simulink model "nav_leha19b"  (R2019b)
settings: Solver=FixedStepDiscrete  StartTime=0.0  StopTime=2500  FixedStep=dT  RelTol=1e-3
values from neighbouring files (symbols this model uses):
  al_gp_M = k    (= 2)    [gnss_data_orig.m]
  al_gp_max = 15    [model_nav_system_flight_simulation_orig.m]
  al_gp_mu = 3.986004418E+14    (= 398600441800000)    [gnss_data_orig.m]
  al_gp_resolution = 1000    [gnss_data_orig.m]
  al_gp_t0 = gnss_strings_2(1,4)    [gnss_data_orig.m]
  dT = 1    [model_nav_system_flight_simulation_orig.m]
  mean_p_ion = 1.3    [model_nav_system_flight_simulation_orig.m]
  mean_p_trop = 0.3    [model_nav_system_flight_simulation_orig.m]
  P0_b_g = zeros(23,23)    [model_nav_system_flight_simulation_orig.m]
  P_b = zeros(21, 21)    [model_nav_system_flight_simulation_orig.m]
  R_a = 6378136    [model_nav_system_flight_simulation_orig.m]
  R_betta = 0.0053171    [model_nav_system_flight_simulation_orig.m]
  R_betta1 = 71 * 10^-7    (= 7.1e-06)    [model_nav_system_flight_simulation_orig.m]
  R_e2 = 0    [model_nav_system_flight_simulation_orig.m]
  R_ge = 9.78049    [model_nav_system_flight_simulation_orig.m]
  R_q = 0.00346775    [model_nav_system_flight_simulation_orig.m]
  R_u = 7.292115*10^(-5)    (= 7.292115e-05)    [model_nav_system_flight_simulation_orig.m]
  sigma_error_acs0 = [SKO_del_n_x SKO_del_n_y SKO_del_n_z]    [model_nav_system_flight_simulation_orig.m]
  sigma_error_DUS0 = [SKO_del_Omega_x SKO_del_Omega_y SKO_del_Omega_z]    [model_nav_system_flight_simulation_orig.m]
  sigma_gnss0 = SKO_p_del_T + SKO_p_del_t + mean_p_ion + mean_p_trop + SKO_p_mnogoluch + SKO_p_noise    (= 5.61)    [model_nav_system_flight_simulation_orig.m]
  SKO_p_del_T = 3    [model_nav_system_flight_simulation_orig.m]
  SKO_p_del_t = 0.01    [model_nav_system_flight_simulation_orig.m]
  SKO_p_mnogoluch = 0.5    [model_nav_system_flight_simulation_orig.m]
  SKO_p_noise = 0.5    [model_nav_system_flight_simulation_orig.m]
  tr_H = flight_mission(3,1)    [model_nav_system_flight_simulation_orig.m]
  W = W'    [model_nav_system_flight_simulation_orig.m]
  X0 = X0'    [model_nav_system_flight_simulation_orig.m]
  X0_b_g = X0_b_g * 0    [model_nav_system_flight_simulation_orig.m]
undefined symbols (not defined in the file or in its folder): al_gp_e, al_gp_health, al_gp_i, al_gp_lan, al_gp_m0, al_gp_sqrt_a, al_gp_w, sigma_error_D_p, sigma_error_D_p1, sigma_gnss0_0, tr_course, tr_fi, tr_la, tr_pitch, tr_roll, tr_V_E, tr_V_H, tr_V_N, tr_X_dgsk, tr_Y_dgsk, tr_Z_dgsk
libraries: simulink_extras x8
(part 3 of 3)

== matlab function nav_leha19b/Алгоритм ССК + UKF/MATLAB Function2 ==
  data: P input; P output; x input; x output; z_k input; F input; H input; G input; R_k input; Q_km1 input; PP output; dt input
function [P, x, PP] = ukf_2(P, x, z_k, F, H, G, R_k, Q_km1, dt)
    
    % раpмерности
    nx = length(x);         
    nq = size(Q_km1, 1);    
    nz = size(R_k, 1);      
    L  = nx + nq + nz;      
    ns = 2 * L + 1;  %число всех сигма точек 

    f = @(X, W) (eye(nx) + F*dt + (F*dt)^2./2) * X + ((eye(nx)+F*dt/2)*G*dt) * W;
    h = @(X, satelite_errors) H * X - satelite_errors; 
	% альфа бетта каппа
    alpha = 0.001;
    beta  = 2;
    kappa = 0;
    
    % вычисленеи весов
    lambda = alpha ^2 * (L + kappa) - L;
    gamma  = sqrt(L + lambda);
    W_m_0  = lambda / (L + lambda);
    W_c_0  = W_m_0 + 1 - alpha^2 + beta;
    W_i    = 1/(2*(L + lambda));
    % дополненная система
    P_a     = blkdiag(P, Q_km1, R_k); %располагаем матрицы по диагонали
    x_a_km1 = [x; zeros(nq, 1); zeros(nz, 1)]; %дополняем вектор состояния
    
    % сигматочечное разложение
%     [u, s] = svd(P_a);
%     gamma_sqrt_P_a = gamma * u * sqrt(s);
%     e = repmat(x_a_km1, 1, L);
%     X_a_km1 = [x_a_km1, ...
%                repmat(x_a_km1, 1, L) + gamma_sqrt_P_a, ...
%                repmat(x_a_km1, 1, L) - gamma_sqrt_P_a];
    gamma_sqrt_P_a = gamma*chol(P_a)';
    e = chol(P_a);
    X_a_km1 = [x_a_km1,...
        repmat(x_a_km1, 1, L) + gamma_sqrt_P_a, ...
        repmat(x_a_km1, 1, L) - gamma_sqrt_P_a,];
    Z_kkm1   = zeros(nz, ns);
    X_x_kkm1 = zeros(nx, ns);
    for sp = 1:ns
        X_x_kkm1(:, sp) = f(X_a_km1(1:nx, sp), X_a_km1(nx+1:nx+nq, sp));            
        Z_kkm1(:, sp)   = h(X_x_kkm1(1:nx, sp), X_a_km1(nx+nq+1:nx+nq+nz, sp));                   
    end
    
    x_kkm1 = W_m_0 * X_x_kkm1(:, 1) + W_i * sum(X_x_kkm1(:, 2:end), 2);
    z_kkm1 = W_m_0 * Z_kkm1(:, 1)   + W_i * sum(Z_kkm1(:, 2:end), 2);

%     X_x_kkm1 = bsxfun(@minus, X_x_kkm1, x_kkm1);
%     Z_kkm1   = bsxfun(@minus, Z_kkm1, z_kkm1);

    X_x_kkm1 = X_x_kkm1 - x_kkm1;
    Z_kkm1   = Z_kkm1 - z_kkm1;
    
    P_kkm1 =   (W_c_0 * X_x_kkm1(:, 1)) * X_x_kkm1(:, 1).' ...
             + W_i * (X_x_kkm1(:, 2:end) * X_x_kkm1(:, 2:end).');

    P_zz =   (W_c_0 * Z_kkm1(:, 1)) * Z_kkm1(:, 1).' ...
           + W_i * (Z_kkm1(:, 2:end) * Z_kkm1(:, 2:end).');
    
    P_xz =   (W_c_0 * X_x_kkm1(:, 1)) * Z_kkm1(:, 1).' ...
           + W_i * (X_x_kkm1(:, 2:end) * Z_kkm1(:, 2:end).');
       
    K = P_xz / P_zz;
    x = x_kkm1 + K * (z_k - Z_kkm1);
    P = P_kkm1 - K * P_zz * K.';
    PP = zeros(21,1);
    for i = 1:1:nx
        PP (i) = sqrt(P(i,i));
    end
end

== matlab function nav_leha19b/Сравнение ССK  и CCK + UKF/MATLAB Function ==
  data: real_data input; plot1 output; estimate input; plot2 output
function [plot1, plot2] = fcn(real_data, estimate)
plot1 = abs(real_data(1));
plot2 = abs(estimate(1));

== matlab function nav_leha19b/Сравнение ССK  и CCK + UKF/MATLAB Function1 ==
  data: real_data input; plot1 output; estimate input; plot2 output
function [plot1, plot2] = fcn(real_data, estimate)
plot1 = abs(real_data(1));
plot2 = abs(estimate(1));

== matlab function nav_leha19b/Алгоритм ЖСК БИНС + ГНСС + UKF/MATLAB Function ==
  settings: updateMethod=DISCRETE  sampleTime=dT
  data: tr_la input; tr_fi input; tr_H input; tr_V_H input; R1 input; ro1 input; H_b_g output size=[2 * al_gp_max, 23]; ro2 input; R_a input; R_e2 input; b_D_p input; pos_x_dgks input; pos_y_dgks input; pos_z_dgks input; b_X_dgsk input; b_Y_dgsk input; b_Z_dgsk input; Omega_id_geogr input; see_flag input; al_gp_max input
function H_b_g = H_b_gp(tr_la, tr_fi, tr_H, tr_V_H, R1, ro1, ro2, R_a, R_e2, b_D_p, pos_x_dgks, pos_y_dgks, pos_z_dgks, b_X_dgsk, b_Y_dgsk, b_Z_dgsk, Omega_id_geogr, see_flag, al_gp_max)
    persistent i j m
    m = sum(see_flag);
    b_la = tr_la;
    b_fi = tr_fi;
    b_H = tr_H;
    b_V_H = tr_V_H;

    Omega_E = Omega_id_geogr(1);
    Omega_N = Omega_id_geogr(2);
    Omega_H = Omega_id_geogr(3);

    i = int8(1);
    j = int8(1);
    
    H_b_g = zeros(2 * al_gp_max, 23);

    while j <= 31
        if see_flag(j) > 0.5
            dR1_db_fi = (R_a * R_e2 * cos(b_fi) * sin(b_fi)) / (( 1 - R_e2 * ((sin(b_fi)) ^ 2)) ^ (3/2));
            
            %Rtp = sin(b_fi) * (R1 + b_H) - cos(b_fi) * dR1_db_fi;
            
            dp_dfi = (1 / b_D_p(j)) * ...
                    ((pos_x_dgks(j) - b_X_dgsk) * (- cos(b_la) * cos(b_fi) * dR1_db_fi + (R1 + b_H) * cos(b_la) * sin(b_fi)) + ...
                     (pos_y_dgks(j) - b_Y_dgsk) * (- sin(b_la) * cos(b_fi) * dR1_db_fi + (R1 + b_H) * sin(b_la) * sin(b_fi)) + ...
                     (pos_z_dgks(j) - b_Z_dgsk) * ( - (1 - R_e2) * sin(b_fi) * dR1_db_fi - ((1 - R_e2) * R1 + b_H) * cos(b_fi)));
            
            dp_dH  = (-1 / b_D_p(j)) * (cos(b_fi) * cos(b_la) * (pos_x_dgks(j) - b_X_dgsk) + ...
                     cos(b_fi) * sin(b_la) * (pos_y_dgks(j) - b_Y_dgsk) + ...
                     sin(b_fi) * (pos_z_dgks(j) - b_Z_dgsk));
                 
            H_b_g(i,1) = (1 / b_D_p(j)) * (sin(b_la) * ... 
                         (pos_x_dgks(j) - b_X_dgsk) - cos(b_la) * (pos_y_dgks(j) - b_Y_dgsk));
            H_b_g(i,2) = (1 / ro1) * dp_dfi;
            H_b_g(i,3) = dp_dH;
            H_b_g(i,20) = -1;
            
            i = i + 1;
            j = j + 1;
        else
            j = j + 1;
        end
    end
    i = int8(m + 1 + (al_gp_max - m));
    j = int8(1);
    while j <= 31
        if see_flag(j) > 0.5
            dp1_db_V_E = (1 / b_D_p(j)) * (sin(b_la) * (pos_x_dgks(j) - b_X_dgsk) - ...
            cos(b_la) * (pos_y_dgks(j) - b_Y_dgsk)); %* del_b_V_E;
        
            dp1_db_V_N = (1 / b_D_p(j)) * (cos(b_la) * sin(b_fi) * (pos_x_dgks(j) - b_X_dgsk) + ...
            sin(b_la) * sin(b_fi) * (pos_y_dgks(j) - b_Y_dgsk) - cos(b_fi) * (pos_z_dgks(j) - b_Z_dgsk));% * del_b_V_N;
            
            dp1_db_V_H = (- 1 / b_D_p(j)) * (cos(b_la) * cos(b_fi) * (pos_x_dgks(j) - b_X_dgsk) + ...
            sin(b_la) * cos(b_fi) * (pos_y_dgks(j) - b_Y_dgsk) + sin(b_fi) * (pos_z_dgks(j) - b_Z_dgsk));% * del_b_V_H;
        
            H_b_g(i,1) = - ((b_V_H / ro2) + Omega_E * tan(b_fi)) * dp1_db_V_E;
            H_b_g(i,2) = - Omega_H * dp1_db_V_E - (b_V_H / ro1) * dp1_db_V_N;
            H_b_g(i,3) = Omega_N * dp1_db_V_E - Omega_E * dp1_db_V_N;
            H_b_g(i,4) = dp1_db_V_E;
            H_b_g(i,5) = dp1_db_V_N;
            H_b_g(i,6) = dp1_db_V_H;
            H_b_g(i,23) = 1;
            
            i = i + 1;
            j = j + 1;
        else
            j = j + 1;
        end
    end

end

== matlab function nav_leha19b/Алгоритм ЖСК БИНС + ГНСС + UKF/MATLAB Function1 ==
  data: rate_X input; Z_b_g_ output size=[30,1]; del_D_p input; D_p input; D1_p input; al_gp_max input
function Z_b_g_ = h(rate_X, del_D_p, D_p, D1_p, al_gp_max)



n = 1;
if n == 1
    Z_b_g_ = zeros(2 * al_gp_max, 1);
    n = n+1;
end
b_D_p = zeros(31,1);
b_D1_p = zeros(31,1);

for i = 1:1:31
    if see_flag(i) > 0.5
        B = [ -sin(tr_la), cos(tr_la), 0;
            -cos(tr_la) * sin(tr_fi), -sin(tr_la) * sin(tr_fi), cos(tr_fi);
            cos(tr_la) * cos(tr_fi), sin(tr_la) * cos(tr_fi), sin(tr_fi)];
        b_V = (B') * [tr_V_E + rate_X(4) - ( (tr_V_H ./ ro2) + Omega_id_geogr(1) .* tan(tr_fi) ) .* rate_X(1) - Omega_id_geogr(3) .* rate_X(2); tr_V_N + rate_X(5) - ( tr_V_H ./ ro1 ) .* rate_X(1); tr_V_H + rate_X(6)];

        b_D_p(i) = sqrt ( (pos_x_dgsk(i) - (tr_H + rate_X(3) + R_a / sqrt(1 - R_e2 * (sin(tr_fi) ^ 2))) * cos(tr_fi + rate_X(2) ./ ro1) * cos(tr_la + rate_X(1) ./ ( ro2 .* cos(tr_fi) ))).^2 + ...
            (pos_y_dgsk(i) - (tr_H + rate_X(3) + R_a / sqrt(1 - R_e2 * (sin(tr_fi) ^ 2))) * cos(tr_fi + rate_X(2) ./ ro1) * sin(tr_la + rate_X(1) ./ ( ro2 .* cos(tr_fi) ))).^2 + ...
            (pos_z_dgsk(i) - ((1 - R_e2) * R_a / sqrt(1 - R_e2 * (sin(tr_fi) ^ 2)) + tr_H + rate_X(3)) * sin(tr_fi + rate_X(2) ./ ro1)).^2);
        b_D1_p(i) = (((pos_x_dgsk(i) - (tr_H + rate_X(3) + R_a / sqrt(1 - R_e2 * (sin(tr_fi) ^ 2))) * cos(tr_fi + rate_X(2) ./ ro1) * cos(tr_la + rate_X(1) ./ ( ro2 .* cos(tr_fi) ))) .* (vel_x_dgsk(i) - b_V(1))) + ...
            ( (pos_y_dgsk(i) - (tr_H + rate_X(3) + R_a / sqrt(1 - R_e2 * (sin(tr_fi) ^ 2))) * cos(tr_fi + rate_X(2) ./ ro1) * sin(tr_la + rate_X(1) ./ ( ro2 .* cos(tr_fi) ))) .* (vel_y_dgsk(i) - b_V(2))) + ...
            ( (pos_z_dgsk(i) - ((1 - R_e2) * R_a / sqrt(1 - R_e2 * (sin(tr_fi) ^ 2)) + tr_H + rate_X(3)) * sin(tr_fi + rate_X(2) ./ ro1)) .* (vel_z_dgsk(i) - b_V(3)))) ./ b_D_p(i);

    else
        b_D_p(i) = NaN;
        b_D1_p(i) = NaN;
    end
end
m = sum(see_flag);
i = 1;
for j = 1:1:31
    if see_flag(j) == 1
        Z_b_g_(i) = b_D_p(j) - D_p(j);
        i = i + 1;
    end
end
i = m + 1 + (al_gp_max - m);
for j = 1:1:31
    if see_flag(j) == 1
        Z_b_g_(i) = b_D1_p(j) - D1_p(j);
        i = i + 1;
    end
end
Z_b_g_ = Z_b_g_ + del_D_p;
end

== matlab function nav_leha19b/Алгоритм ЖСК БИНС + ГНСС/MATLAB Function2 ==
  data: X_diff input; X_feedback output; X_b input
function X_feedback = fcn(X_diff, X_b)
X_feedback = X_b;
X_feedback(1:2) = X_diff(1:2);
X_feedback(4:5) = X_diff(4:5);
X_feedback(7:21) = X_diff(7:21);
end

== matlab function nav_leha19b/Алгоритм ЖСК БИНС + ГНСС + UKF/MATLAB Function2 ==
  data: X_diff input; X_b input; X_feedback output
function X_feedback = fcn(X_diff, X_b)
X_feedback = X_b;
X_feedback(1:2) = X_diff(1:2);
X_feedback(4:5) = X_diff(4:5);
X_feedback(7:21) = X_diff(7:21);
end

== matlab function nav_leha19b/Алгоритм ЖСК БИНС + ГНСС + UKF/MATLAB Function3 ==
  data: F_b input size=[21,21]; G_b input; F_b_g output size=[23,23]; G_b_g output
function [F_b_g, G_b_g]  = fcn(F_b, G_b)

    F_b_g = zeros(23,23);
    F_b_g(1:21, 1:21) = F_b;

    G_b_g = zeros(23,6);
    G_b_g(1:21, 1:6) = G_b;
    
end

== matlab function nav_leha19b/pseudorange/MATLAB Function4 ==
  data: El input; HDOP output; az input; see_flag input; VDOP output; PDOP output; TDOP output; al_gp_max input
function [HDOP, VDOP, PDOP, TDOP] = fcn(El, az, see_flag, al_gp_max)
DOP_A = zeros(al_gp_max,4);

persistent i k
k = 1;
for i = 1:31
    if see_flag(i) > 0.5
        DOP_A(k,1) = - cos(El(i))*cos(az(i));
        DOP_A(k,2) = - cos(El(i))*sin(az(i));
        DOP_A(k,3) = - sin(El(i));
        DOP_A(k,4) = 1;
        k = k + 1;
    end
end
DOP_H = (DOP_A'*DOP_A)^(-1);
HDOP = sqrt(DOP_H(1,1) + DOP_H(2,2));
VDOP = sqrt(DOP_H(3,3));
PDOP = sqrt(DOP_H(1,1) + DOP_H(2,2) + DOP_H(3,3));
TDOP = sqrt(DOP_H(4,4));

== matlab function nav_leha19b/Алгоритм ЖСК БИНС + ГНСС + UKF/MATLAB Function4 ==
  settings: updateMethod=DISCRETE  sampleTime=dT
  data: P input; P output; x input; z_k input; F input; G input; R_k input; Q_km1 input; dt input; x output; x_21 output size=21; PP output size=[23]; x12 output size=2; pos_x_dgsk input; pos_y_dgsk input; pos_z_dgsk input; vel_x_dgsk input; vel_y_dgsk input; vel_z_dgsk input; see_flag input; tr_fi input; tr_la input; tr_H input; tr_V_E input; tr_V_N input; tr_V_H input; ro1 input; ro2 input; R_a input; R_e2 input; al_gp_max input; D_p input; Omega_id_geogr input; D1_p input; e output size=[1,1]; l output size=[1,1]
function [P, x, x_21, PP, x12, e, l] = ukf_2(P, x, z_k, F, G, R_k, Q_km1, dt, pos_x_dgsk, pos_y_dgsk, pos_z_dgsk, vel_x_dgsk, vel_y_dgsk, vel_z_dgsk, see_flag, tr_fi, tr_la, tr_H, tr_V_E, tr_V_N, tr_V_H, ro1, ro2, R_a, R_e2, al_gp_max, D_p, Omega_id_geogr, D1_p)

    function Z_b_g_ = h(rate_X, del_D_p)
        n = 1;
        if n == 1
            Z_b_g_ = zeros(2 * al_gp_max, 1);
            n = n+1;
        end
        b_D_p = zeros(31,1);
        b_D1_p = zeros(31,1);

        for i = 1:1:31
            if see_flag(i) > 0.5
                B = [ -sin(tr_la), cos(tr_la), 0;
                    -cos(tr_la) * sin(tr_fi), -sin(tr_la) * sin(tr_fi), cos(tr_fi);
                    cos(tr_la) * cos(tr_fi), sin(tr_la) * cos(tr_fi), sin(tr_fi)];
                b_V = (B') * [tr_V_E + rate_X(4) - ( (tr_V_H ./ ro2) + Omega_id_geogr(1) .* tan(tr_fi) ) .* rate_X(1) - Omega_id_geogr(3) .* rate_X(2); tr_V_N + rate_X(5) - ( tr_V_H ./ ro1 ) .* rate_X(1); tr_V_H + rate_X(6)];

                b_D_p(i) = sqrt ( (pos_x_dgsk(i) - (tr_H + rate_X(3) + R_a / sqrt(1 - R_e2 * (sin(tr_fi) ^ 2))) * cos(tr_fi + rate_X(2) ./ ro1) * cos(tr_la + rate_X(1) ./ ( ro2 .* cos(tr_fi) ))).^2 + ...
                    (pos_y_dgsk(i) - (tr_H + rate_X(3) + R_a / sqrt(1 - R_e2 * (sin(tr_fi) ^ 2))) * cos(tr_fi + rate_X(2) ./ ro1) * sin(tr_la + rate_X(1) ./ ( ro2 .* cos(tr_fi) ))).^2 + ...
                    (pos_z_dgsk(i) - ((1 - R_e2) * R_a / sqrt(1 - R_e2 * (sin(tr_fi) ^ 2)) + tr_H + rate_X(3)) * sin(tr_fi + rate_X(2) ./ ro1)).^2);
                b_D1_p(i) = (((pos_x_dgsk(i) - (tr_H + rate_X(3) + R_a / sqrt(1 - R_e2 * (sin(tr_fi) ^ 2))) * cos(tr_fi + rate_X(2) ./ ro1) * cos(tr_la + rate_X(1) ./ ( ro2 .* cos(tr_fi) ))) .* (vel_x_dgsk(i) - b_V(1))) + ...
                ( (pos_y_dgsk(i) - (tr_H + rate_X(3) + R_a / sqrt(1 - R_e2 * (sin(tr_fi) ^ 2))) * cos(tr_fi + rate_X(2) ./ ro1) * sin(tr_la + rate_X(1) ./ ( ro2 .* cos(tr_fi) ))) .* (vel_y_dgsk(i) - b_V(2))) + ...
                ( (pos_z_dgsk(i) - ((1 - R_e2) * R_a / sqrt(1 - R_e2 * (sin(tr_fi) ^ 2)) + tr_H + rate_X(3)) * sin(tr_fi + rate_X(2) ./ ro1)) .* (vel_z_dgsk(i) - b_V(3)))) ./ b_D_p(i);

            else
                b_D_p(i) = NaN;
                b_D1_p(i) = NaN;
            end
        end
        m = sum(see_flag);
        i = 1;
        for j = 1:1:31
            if see_flag(j) == 1
                Z_b_g_(i) = b_D_p(j) - D_p(j);
                i = i + 1;
            end
        end
        i = m + 1 + (al_gp_max - m);
        for j = 1:1:31
            if see_flag(j) == 1
                Z_b_g_(i) = b_D1_p(j) - D1_p(j);
                i = i + 1;
            end
        end
       Z_b_g_ = Z_b_g_ + del_D_p;
    end

% размерности
nx = length(x);
nq = size(Q_km1, 1);
nz = size(R_k, 1);
L  = nx + nq + nz;
ns = 2 * L + 1;  %число всех сигма точек

f = @(X, W) (eye(nx) + F*dt + (F*dt)^2./2) * X + ((eye(nx)+F*dt/2)*G*dt) * W;
%     h = @(X, satelite_errors) H * X;% - satelite_errors;
% альфа бетта каппа
alpha = 0.001;
beta  = 2;
kappa = 3 - nx;

% вычисленеи весов
lambda = alpha ^2 * (L + kappa) - L;
gamma  = sqrt(L + lambda);
W_m_0  = lambda / (L + lambda);
W_c_0  = W_m_0 + 1 - alpha^2 + beta;
W_i    = 1/(2*(L + lambda));
% дополненная система
P_a     = blkdiag(P, Q_km1, R_k); %располагаем матрицы по диагонали
x_a_km1 = [x; zeros(nq, 1); zeros(nz, 1)]; %дополняем вектор состояния

gamma_sqrt_P_a = gamma*chol(P_a)';
X_a_km1 = [x_a_km1,...
    repmat(x_a_km1, 1, L) + gamma_sqrt_P_a, ...
    repmat(x_a_km1, 1, L) - gamma_sqrt_P_a,];
Z_kkm1   = zeros(nz, ns);
X_x_kkm1 = zeros(nx, ns);
for sp = 1:ns
    X_x_kkm1(:, sp) = f(X_a_km1(1:nx, sp), X_a_km1(nx+1:nx+nq, sp));
    Z_kkm1(:, sp)   = h(X_x_kkm1(1:nx, sp), X_a_km1(nx+nq+1:nx+nq+nz, sp));
end

x_kkm1 = W_m_0 * X_x_kkm1(:, 1) + W_i * sum(X_x_kkm1(:, 2:end), 2);
z_kkm1 = W_m_0 * Z_kkm1(:, 1)   + W_i * sum(Z_kkm1(:, 2:end), 2);

%     X_x_kkm1 = bsxfun(@minus, X_x_kkm1, x_kkm1);
%     Z_kkm1   = bsxfun(@minus, Z_kkm1, z_kkm1);

X_x_kkm1 = X_x_kkm1 - x_kkm1;
Z_kkm1   = Z_kkm1 - z_kkm1;

P_kkm1 =   (W_c_0 * X_x_kkm1(:, 1)) * X_x_kkm1(:, 1).' ...
    + W_i * (X_x_kkm1(:, 2:end) * X_x_kkm1(:, 2:end).');

P_zz =   (W_c_0 * Z_kkm1(:, 1)) * Z_kkm1(:, 1).' ...
    + W_i * (Z_kkm1(:, 2:end) * Z_kkm1(:, 2:end).');

P_xz =   (W_c_0 * X_x_kkm1(:, 1)) * Z_kkm1(:, 1).' ...
    + W_i * (X_x_kkm1(:, 2:end) * Z_kkm1(:, 2:end).');

K = P_xz / P_zz;
e = z_k(1,1);
size(e);

l = z_kkm1(1,1);
size(l);
x = x_kkm1 + K * (z_k - z_kkm1);
P = P_kkm1 - K * P_zz * K.';
PP = zeros(nx,1);
for ii = 1:1:nx
    PP(ii) = sqrt(P(ii,ii));
end
x_21 = x(1:21);
x12 = x(1:2);
% ZZ = h(X, 0);
% size(ZZ)
end

== matlab function nav_leha19b/Алгоритм ЖСК БИНС + ГНСС + UKF/MATLAB Function5 ==
  settings: updateMethod=DISCRETE  sampleTime=dT
  data: sigma_error_D_p input; Rv_b_g output size=[2 * al_gp_max, 2 * al_gp_max]; sigma_error_D_p1 input; sigma_error_DUS input; sigma_error_acs input; SKO_gnss0 input; sigma_error_DUS0 input; sigma_error_acs0 input; dt input; Q_W output; T input; see_flag input; al_gp_max input
function [Rv_b_g, Q_W] = fcn(sigma_error_D_p, sigma_error_D_p1, sigma_error_DUS, sigma_error_acs, SKO_gnss0, sigma_error_DUS0, sigma_error_acs0, dt, T, see_flag, al_gp_max)

== matlab function nav_leha19b/Алгоритм ЖСК БИНС + ГНСС + UKF/MATLAB Function6 ==
  data: rate_X_feedback output; X_b input; rate_X input
function rate_X_feedback = fcn(X_b, rate_X)
rate_X_feedback = rate_X;

% rate_X_feedback(1:21) = X_b;
% rate_X_feedback(1:2) = 0;
% rate_X_feedback(4:5) = 0;
% rate_X_feedback(22:23) = rate_X(22:23);
end

== matlab function nav_leha19b/Сравнение ССK  и CCK + UKF1/MATLAB Function ==
  data: real_data input; plot1 output; estimate input; plot2 output
function [plot1, plot2] = fcn(real_data, estimate)
plot1 = (real_data(4));
plot2 = (estimate(4));

== matlab function nav_leha19b/Сравнение ССK  и CCK + UKF1/MATLAB Function1 ==
  data: real_data input; plot1 output; estimate input; plot2 output
function [plot1, plot2] = fcn(real_data, estimate)
plot1 = (real_data(4));
plot2 = (estimate(4));

== matlab function nav_leha19b/Сравнение ССK  и CCK + UKF1/MATLAB Function2 ==
  data: real_data input; EKF output; estimate input; UFK output
function [EKF, UFK] = fcn(real_data, estimate)
EKF = (real_data(1));
UFK = (estimate(1));

== matlab function nav_leha19b/Алгоритм ЖСК БИНС + ГНСС/MATLAB Function6 ==
  data: rate_X_feedback output; X_b input; rate_X input
function rate_X_feedback = fcn(X_b, rate_X)
rate_X_feedback = rate_X;

rate_X_feedback(1:21) = X_b;
rate_X_feedback(1:2) = 0;
rate_X_feedback(4:5) = 0;
rate_X_feedback(22:23) = rate_X(22:23);
end

== matlab function nav_leha19b/Сравнение ССK  и CCK + UKF1/MATLAB Function3 ==
  data: real_data input; plot1 output; estimate input; plot2 output
function [plot1, plot2] = fcn(real_data, estimate)
plot1 = (real_data(1));
plot2 = (estimate(1));

== matlab function nav_leha19b/MATLAB Function7 ==
  settings: updateMethod=DISCRETE  sampleTime=dT
  data: rate_X input; Z_b_g_ output size=[2*al_gp_max,1]; pos_x_dgsk input; pos_y_dgsk input; pos_z_dgsk input; see_flag input; tr_fi input; tr_la input; tr_H input; ro1 input; ro2 input; R_a input; R_e2 input; al_gp_max input; D_p input
function Z_b_g_ = fcn(rate_X, pos_x_dgsk, pos_y_dgsk, pos_z_dgsk, see_flag, tr_fi, tr_la, tr_H, ro1, ro2, R_a, R_e2, al_gp_max, D_p)
        n = 1;
        if n == 1
            Z_b_g_ = zeros(2 * al_gp_max, 1);
            n = n+1;
        end
        b_D_p = zeros(31,1);
        b_D1_p = zeros(31,1);
      
        for i = 1:1:31
            if see_flag(i) > 0.5
                
                b_D_p(i) = sqrt ( (pos_x_dgsk(i) - (tr_H + rate_X(3) + R_a / sqrt(1 - R_e2 * (sin(tr_fi) ^ 2))) * cos(tr_fi + rate_X(2) ./ ro1) * cos(tr_la + rate_X(1) ./ ( ro2 .* cos(tr_fi) ))).^2 + ...
                    (pos_y_dgsk(i) - (tr_H + rate_X(3) + R_a / sqrt(1 - R_e2 * (sin(tr_fi) ^ 2))) * cos(tr_fi + rate_X(2) ./ ro1) * sin(tr_la + rate_X(1) ./ ( ro2 .* cos(tr_fi) ))).^2 + ...
                    (pos_z_dgsk(i) - ((1 - R_e2) * R_a / sqrt(1 - R_e2 * (sin(tr_fi) ^ 2)) + tr_H + rate_X(3)) * sin(tr_fi + rate_X(2) ./ ro1)).^2 );
                b_D1_p(i) = 0; %(((pos_x_dgsk(i) - b_X_dgsk) .* (vel_x_dgsk(i) - b_V_1)) + ...
                            %( (pos_y_dgsk(i) - b_Y_dgsk) .* (vel_y_dgsk(i) - b_V_2)) + ...
                            %( (pos_z_dgsk(i) - b_Z_dgsk) .* (vel_z_dgsk(i) - b_V_3))) ./ b_D_p(i);
                            
            else
                b_D_p(i) = NaN;
                b_D1_p(i) = NaN;
            end
        end
        m = sum(see_flag);
        i = 1;
        for j = 1:1:31
            if see_flag(j) == 1
                Z_b_g_(i) = b_D_p(j) - D_p(j);
                i = i + 1;
            end
        end
        i = m + 1 + (al_gp_max - m);
        for j = 1:1:31
            if see_flag(j) == 1
                Z_b_g_(i) = 0; %b_D1_p(j) - D1_p(j);
                i = i + 1;
            end
        end
    end

== matlab function nav_leha19b/Алгоритм ЖСК БИНС + ГНСС + UKF/MATLAB Function7 ==
  settings: updateMethod=DISCRETE  sampleTime=dT
  data: rate_X input; Z_b_g_ output size=[2*al_gp_max,1]; pos_x_dgsk input; pos_y_dgsk input; pos_z_dgsk input; see_flag input; tr_fi input; tr_la input; tr_H input; ro1 input; ro2 input; R_a input; R_e2 input; al_gp_max input; D_p input; del_D_p input
function Z_b_g_ = h(rate_X, pos_x_dgsk, pos_y_dgsk, pos_z_dgsk, see_flag, tr_fi, tr_la, tr_H, ro1, ro2, R_a, R_e2, al_gp_max, D_p, del_D_p)
        n = 1;
        if n == 1
            Z_b_g_ = zeros(2 * al_gp_max, 1);
            n = n+1;
        end
        b_D_p = zeros(31,1);
        b_D1_p = zeros(31,1);
      
        for i = 1:1:31
            if see_flag(i) > 0.5
                
                b_D_p(i) = sqrt ( (pos_x_dgsk(i) - (tr_H + rate_X(3) + R_a / sqrt(1 - R_e2 * (sin(tr_fi) ^ 2))) * cos(tr_fi + rate_X(2) ./ ro1) * cos(tr_la + rate_X(1) ./ ( ro2 .* cos(tr_fi) ))).^2 + ...
                    (pos_y_dgsk(i) - (tr_H + rate_X(3) + R_a / sqrt(1 - R_e2 * (sin(tr_fi) ^ 2))) * cos(tr_fi + rate_X(2) ./ ro1) * sin(tr_la + rate_X(1) ./ ( ro2 .* cos(tr_fi) ))).^2 + ...
                    (pos_z_dgsk(i) - ((1 - R_e2) * R_a / sqrt(1 - R_e2 * (sin(tr_fi) ^ 2)) + tr_H + rate_X(3)) * sin(tr_fi + rate_X(2) ./ ro1)).^2 ) + del_D_p(i);
                b_D1_p(i) = 0; %(((pos_x_dgsk(i) - b_X_dgsk) .* (vel_x_dgsk(i) - b_V_1)) + ...
                            %( (pos_y_dgsk(i) - b_Y_dgsk) .* (vel_y_dgsk(i) - b_V_2)) + ...
                            %( (pos_z_dgsk(i) - b_Z_dgsk) .* (vel_z_dgsk(i) - b_V_3))) ./ b_D_p(i);
                            
            else
                b_D_p(i) = NaN;
                b_D1_p(i) = NaN;
            end
        end
        m = sum(see_flag);
        i = 1;
        for j = 1:1:31
            if see_flag(j) == 1
                Z_b_g_(i) = b_D_p(j) - D_p(j);
                i = i + 1;
            end
        end
        i = m + 1 + (al_gp_max - m);
        for j = 1:1:31
            if see_flag(j) == 1
                Z_b_g_(i) = 0; %b_D1_p(j) - D1_p(j);
                i = i + 1;
            end
        end
    end

== matlab function nav_leha19b/Сравнение ССK  и CCK + UKF1/MATLAB Function4 ==
  data: real_data input; plot1 output; estimate input; plot2 output
function [plot1, plot2] = fcn(real_data, estimate)
plot1 = (real_data(2));
plot2 = (estimate(2));

== matlab function nav_leha19b/Сравнение ССK  и CCK + UKF1/MATLAB Function5 ==
  data: real_data input; plot1 output; estimate input; plot2 output
function [plot1, plot2] = fcn(real_data, estimate)
plot1 = (real_data(2));
plot2 = (estimate(2));

== matlab function nav_leha19b/Сравнение ССK  и CCK + UKF1/MATLAB Function6 ==
  data: real_data input; plot1 output; estimate input; plot2 output
function [plot1, plot2] = fcn(real_data, estimate)
plot1 = (real_data(5));
plot2 = (estimate(5));

== matlab function nav_leha19b/Сравнение ССK  и CCK + UKF1/MATLAB Function7 ==
  data: real_data input; plot1 output; estimate input; plot2 output
function [plot1, plot2] = fcn(real_data, estimate)
plot1 = (real_data(5));
plot2 = (estimate(5));

== matlab function nav_leha19b/Алгоритм ССК/MATLAB Function2 ==
  data: rate_X input; rate_X_ output
function rate_X_ = fcn(rate_X)
rate_X_ = rate_X
rate_X_ (1:6) = 0;
end

== matlab function nav_leha19b/Алгоритм ССК/MATLAB Function3 ==
  data: diff_X input; X_CCK_feedback output
function X_CCK_feedback = fcn(diff_X)
X_CCK_feedback = zeros(21,1);
X_CCK_feedback(1:6) = diff_X(1:6);
end
